simulink model "Four_Robots_Swarm"  (R2021a)
settings: Solver=FixedStepAuto  StartTime=0.0  StopTime=inf  FixedStep=0.01  RelTol=1e-3  EnableMultiTasking=on
model workspace (MAT data in the model file):
  SL_ROS_VariableLengthArrays_MaxSizes : object (value not decoded)
undefined symbols (not defined in the file or in its folder): Angular, DistanceGoal, L, Linear, PP, theta, Way1, Way2, Way3, Way4
libraries: robotlib x17, robotalgslib x8
(part 2 of 2)

== system Four_Robots_Swarm/Swarm/TurtleBot2/ Avoiding Obstacles/Path Following ==
  SteeringDirection : Inport
  AngularVelocity : Inport  Port=2
  Action Port : ActionPort  ActionPortLabel=else
  Compute Angular Velocity : MATLAB Function  TreatAsAtomicUnit=on
  Constant : Constant  Value=0
  MaxAngularVelocity : Constant  Value=1.82
  Subtract : Sum  Inputs=+-
  dV : Outport  VectorParamsAs1DForOutWhenUnconnected=off
  dW : Outport  Port=2  VectorParamsAs1DForOutWhenUnconnected=off
  wires:
  AngularVelocity/1 -> Subtract/2
  Compute Angular Velocity/1(w) -> Subtract/1
  Subtract/1 -> dW/1
  SteeringDirection/1 -> Compute Angular Velocity/1(steeringDir)
  MaxAngularVelocity/1 -> Compute Angular Velocity/2(wMax)
  Constant/1 -> dV/1

== system Four_Robots_Swarm/Swarm/TurtleBot2/ Avoiding Obstacles/Recovery ==
  LinearVelocity : Inport
  AngularVelocity_comp : Inport  Port=2
  AngularVelocity : Inport  Port=3
  Action Port : ActionPort  ActionPortLabel=if(u1 == 1)
  Gain : Gain  Gain=-1
  Subtract : Sum  Inputs=|+-
  dV : Outport  VectorParamsAs1DForOutWhenUnconnected=off
  dW : Outport  Port=2  VectorParamsAs1DForOutWhenUnconnected=off
  wires:
  Subtract/1 -> dW/1
  AngularVelocity/1 -> Subtract/2
  Gain/1 -> dV/1
  LinearVelocity/1 -> Gain/1
  AngularVelocity_comp/1 -> Subtract/1

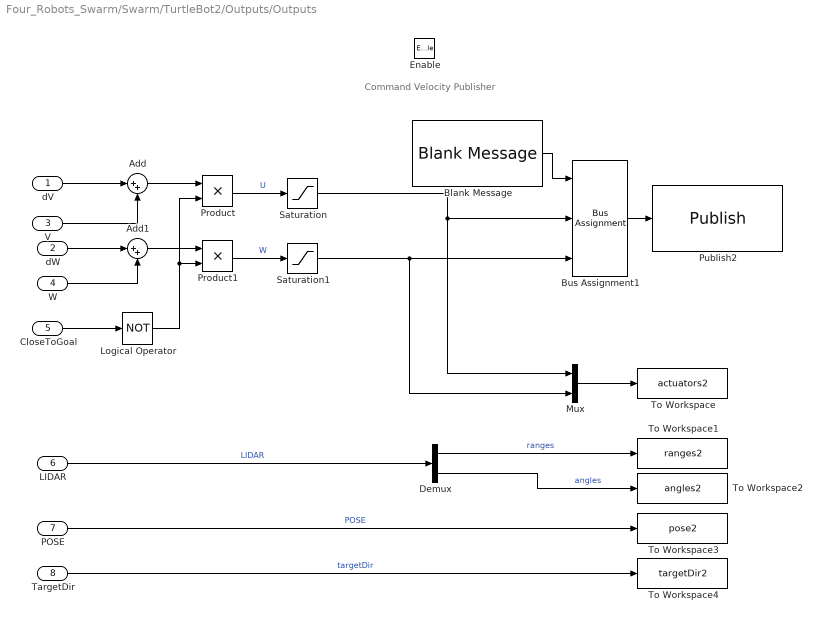
== system Four_Robots_Swarm/Swarm/TurtleBot2/Outputs/Outputs ==
  note: Command Velocity Publisher
  dV : Inport
  dW : Inport  Port=2
  V : Inport  Port=3
  W : Inport  Port=4
  CloseToGoal : Inport  Port=5
  LIDAR : Inport  Port=6
  POSE : Inport  Port=7
  TargetDir : Inport  Port=8
  Enable : EnablePort
  Add : Sum  Inputs=|++
  Add1 : Sum  Inputs=|++
  Blank Message : robotlib/Blank Message  messageClass=Message  entityType=geometry_msgs/Twist  messageType=geometry_msgs/Twist  SampleTime=inf  legacyBusStruct=off
  Bus Assignment1 : BusAssignment  DialogController=Simulink.DDGSource_BusAssignment  AssignedSignals=Linear.X,Angular.Z
  Demux : Demux  Outputs=2
  Logical Operator : Logic  Operator=NOT  AllPortsSameDT=off  OutDataTypeStr=boolean
  Mux : Mux  Inputs=2
  Product : Product
  Product1 : Product
  Publish2 : robotlib/Publish  topicSource=Select from ROS network  topic=/robot2/cmd_vel  messageType=geometry_msgs/Twist  legacyBusStruct=off  messageQueueLength=105
  Saturation : Saturate  UpperLimit=PP.DesiredLinearVelocity  LowerLimit=-PP.DesiredLinearVelocity
  Saturation1 : Saturate  UpperLimit=PP.MaxAngularVelocity  LowerLimit=-PP.MaxAngularVelocity
  To Workspace : ToWorkspace  VariableName=actuators2  SaveFormat=Structure With Time  SampleTime=0.01
      settings: Decimation=2
  To Workspace1 : ToWorkspace  VariableName=ranges2  SaveFormat=Structure With Time  SampleTime=0.01
      settings: Decimation=2
  To Workspace2 : ToWorkspace  VariableName=angles2  SaveFormat=Structure With Time  SampleTime=0.01
      settings: Decimation=2
  To Workspace3 : ToWorkspace  VariableName=pose2  SaveFormat=Structure With Time  SampleTime=0.01
      settings: Decimation=2
  To Workspace4 : ToWorkspace  VariableName=targetDir2  SaveFormat=Structure With Time  SampleTime=0.01
      settings: Decimation=2
  wires:
  V/1 -> Add/2
  W/1 -> Add1/2
  dV/1 -> Add/1
  dW/1 -> Add1/1
  CloseToGoal/1 -> Logical Operator/1
  Add/1 -> Product/1
  Add1/1 -> Product1/1
  Blank Message/1 -> Bus Assignment1/1
  Bus Assignment1/1 -> Publish2/1
  Logical Operator/1 -> Product1/2, Product/2
  Mux/1 -> To Workspace/1
  Product/1 -> Saturation/1  "U"
  Saturation/1 -> Mux/1, Bus Assignment1/2
  Product1/1 -> Saturation1/1  "W"
  Saturation1/1 -> Mux/2, Bus Assignment1/3
  TargetDir/1 -> To Workspace4/1  "targetDir"
  Demux/2 -> To Workspace2/1  "angles"
  LIDAR/1 -> Demux/1  "LIDAR"
  POSE/1 -> To Workspace3/1  "POSE"
  Demux/1 -> To Workspace1/1  "ranges"

== system Four_Robots_Swarm/Swarm/TurtleBot2/Subsystem/Enabled Subsystem ==
  WAY : Inport
  DATA : Inport  Port=2
  Enable : EnablePort
  MATLAB Function2 : MATLAB Function  TreatAsAtomicUnit=on
  I : Outport
  wires:
  WAY/1 -> MATLAB Function2/1(WAY)
  DATA/1 -> MATLAB Function2/2(DATA)
  MATLAB Function2/1(I) -> I/1

== system Four_Robots_Swarm/Swarm/TurtleBot3/ Avoiding Obstacles/Path Following ==
  SteeringDirection : Inport
  AngularVelocity : Inport  Port=2
  Action Port : ActionPort  ActionPortLabel=else
  Compute Angular Velocity : MATLAB Function  TreatAsAtomicUnit=on
  Constant : Constant  Value=0
  MaxAngularVelocity : Constant  Value=1.82
  Subtract : Sum  Inputs=+-
  dV : Outport  VectorParamsAs1DForOutWhenUnconnected=off
  dW : Outport  Port=2  VectorParamsAs1DForOutWhenUnconnected=off
  wires:
  AngularVelocity/1 -> Subtract/2
  Compute Angular Velocity/1(w) -> Subtract/1
  Subtract/1 -> dW/1
  SteeringDirection/1 -> Compute Angular Velocity/1(steeringDir)
  MaxAngularVelocity/1 -> Compute Angular Velocity/2(wMax)
  Constant/1 -> dV/1

== system Four_Robots_Swarm/Swarm/TurtleBot3/ Avoiding Obstacles/Recovery ==
  LinearVelocity : Inport
  AngularVelocity_comp : Inport  Port=2
  AngularVelocity : Inport  Port=3
  Action Port : ActionPort  ActionPortLabel=if(u1 == 1)
  Gain : Gain  Gain=-1
  Subtract : Sum  Inputs=|+-
  dV : Outport  VectorParamsAs1DForOutWhenUnconnected=off
  dW : Outport  Port=2  VectorParamsAs1DForOutWhenUnconnected=off
  wires:
  Subtract/1 -> dW/1
  AngularVelocity/1 -> Subtract/2
  Gain/1 -> dV/1
  LinearVelocity/1 -> Gain/1
  AngularVelocity_comp/1 -> Subtract/1

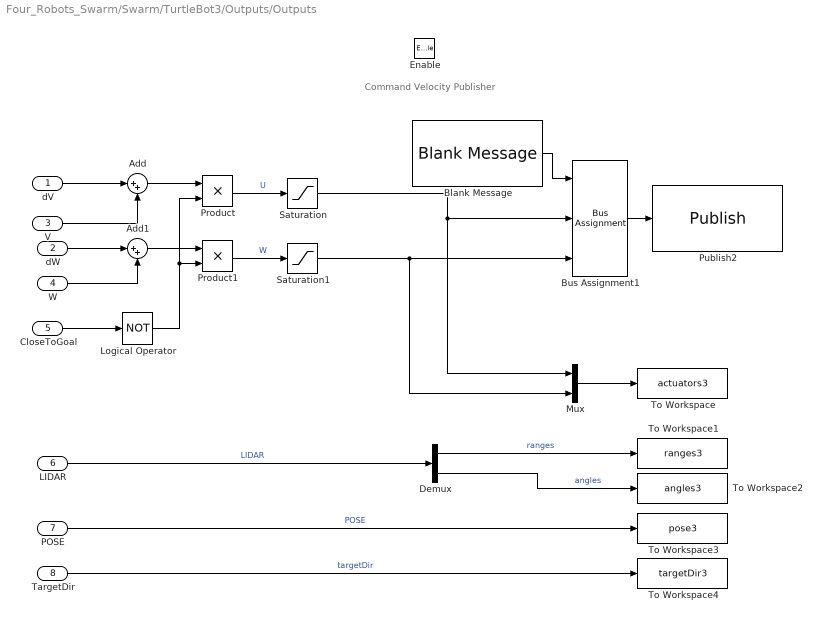
== system Four_Robots_Swarm/Swarm/TurtleBot3/Outputs/Outputs ==
  note: Command Velocity Publisher
  dV : Inport
  dW : Inport  Port=2
  V : Inport  Port=3
  W : Inport  Port=4
  CloseToGoal : Inport  Port=5
  LIDAR : Inport  Port=6
  POSE : Inport  Port=7
  TargetDir : Inport  Port=8
  Enable : EnablePort
  Add : Sum  Inputs=|++
  Add1 : Sum  Inputs=|++
  Blank Message : robotlib/Blank Message  messageClass=Message  entityType=geometry_msgs/Twist  messageType=geometry_msgs/Twist  SampleTime=inf  legacyBusStruct=off
  Bus Assignment1 : BusAssignment  DialogController=Simulink.DDGSource_BusAssignment  AssignedSignals=Linear.X,Angular.Z
  Demux : Demux  Outputs=2
  Logical Operator : Logic  Operator=NOT  AllPortsSameDT=off  OutDataTypeStr=boolean
  Mux : Mux  Inputs=2
  Product : Product
  Product1 : Product
  Publish2 : robotlib/Publish  topicSource=Select from ROS network  topic=/robot3/cmd_vel  messageType=geometry_msgs/Twist  legacyBusStruct=off  messageQueueLength=105
  Saturation : Saturate  UpperLimit=PP.DesiredLinearVelocity  LowerLimit=-PP.DesiredLinearVelocity
  Saturation1 : Saturate  UpperLimit=PP.MaxAngularVelocity  LowerLimit=-PP.MaxAngularVelocity
  To Workspace : ToWorkspace  VariableName=actuators3  SaveFormat=Structure With Time  SampleTime=0.01
      settings: Decimation=2
  To Workspace1 : ToWorkspace  VariableName=ranges3  SaveFormat=Structure With Time  SampleTime=0.01
      settings: Decimation=2
  To Workspace2 : ToWorkspace  VariableName=angles3  SaveFormat=Structure With Time  SampleTime=0.01
      settings: Decimation=2
  To Workspace3 : ToWorkspace  VariableName=pose3  SaveFormat=Structure With Time  SampleTime=0.01
      settings: Decimation=2
  To Workspace4 : ToWorkspace  VariableName=targetDir3  SaveFormat=Structure With Time  SampleTime=0.01
      settings: Decimation=2
  wires:
  V/1 -> Add/2
  W/1 -> Add1/2
  dV/1 -> Add/1
  dW/1 -> Add1/1
  CloseToGoal/1 -> Logical Operator/1
  Add/1 -> Product/1
  Add1/1 -> Product1/1
  Blank Message/1 -> Bus Assignment1/1
  Bus Assignment1/1 -> Publish2/1
  Logical Operator/1 -> Product1/2, Product/2
  Mux/1 -> To Workspace/1
  Product/1 -> Saturation/1  "U"
  Saturation/1 -> Mux/1, Bus Assignment1/2
  Product1/1 -> Saturation1/1  "W"
  Saturation1/1 -> Mux/2, Bus Assignment1/3
  TargetDir/1 -> To Workspace4/1  "targetDir"
  Demux/2 -> To Workspace2/1  "angles"
  LIDAR/1 -> Demux/1  "LIDAR"
  POSE/1 -> To Workspace3/1  "POSE"
  Demux/1 -> To Workspace1/1  "ranges"

== system Four_Robots_Swarm/Swarm/TurtleBot3/Subsystem/Enabled Subsystem ==
  WAY : Inport
  DATA : Inport  Port=2
  Enable : EnablePort
  MATLAB Function2 : MATLAB Function  TreatAsAtomicUnit=on
  I : Outport
  wires:
  WAY/1 -> MATLAB Function2/1(WAY)
  DATA/1 -> MATLAB Function2/2(DATA)
  MATLAB Function2/1(I) -> I/1

== system Four_Robots_Swarm/Swarm/TurtleBot4/ Avoiding Obstacles/Path Following ==
  SteeringDirection : Inport
  AngularVelocity : Inport  Port=2
  Action Port : ActionPort  ActionPortLabel=else
  Compute Angular Velocity : MATLAB Function  TreatAsAtomicUnit=on
  Constant : Constant  Value=0
  MaxAngularVelocity : Constant  Value=1.82
  Subtract : Sum  Inputs=+-
  dV : Outport  VectorParamsAs1DForOutWhenUnconnected=off
  dW : Outport  Port=2  VectorParamsAs1DForOutWhenUnconnected=off
  wires:
  AngularVelocity/1 -> Subtract/2
  Compute Angular Velocity/1(w) -> Subtract/1
  Subtract/1 -> dW/1
  SteeringDirection/1 -> Compute Angular Velocity/1(steeringDir)
  MaxAngularVelocity/1 -> Compute Angular Velocity/2(wMax)
  Constant/1 -> dV/1

== system Four_Robots_Swarm/Swarm/TurtleBot4/ Avoiding Obstacles/Recovery ==
  LinearVelocity : Inport
  AngularVelocity_comp : Inport  Port=2
  AngularVelocity : Inport  Port=3
  Action Port : ActionPort  ActionPortLabel=if(u1 == 1)
  Gain : Gain  Gain=-1
  Subtract : Sum  Inputs=|+-
  dV : Outport  VectorParamsAs1DForOutWhenUnconnected=off
  dW : Outport  Port=2  VectorParamsAs1DForOutWhenUnconnected=off
  wires:
  Subtract/1 -> dW/1
  AngularVelocity/1 -> Subtract/2
  Gain/1 -> dV/1
  LinearVelocity/1 -> Gain/1
  AngularVelocity_comp/1 -> Subtract/1

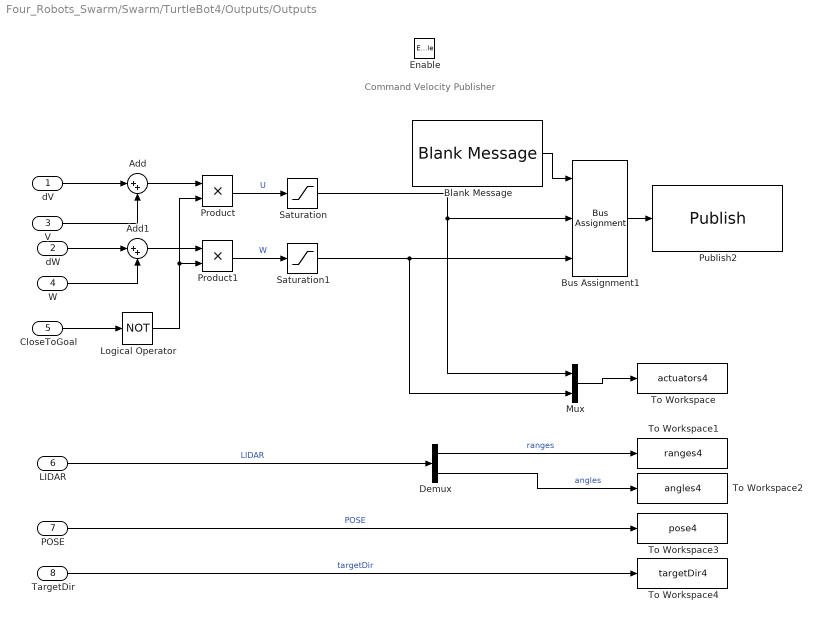
== system Four_Robots_Swarm/Swarm/TurtleBot4/Outputs/Outputs ==
  note: Command Velocity Publisher
  dV : Inport
  dW : Inport  Port=2
  V : Inport  Port=3
  W : Inport  Port=4
  CloseToGoal : Inport  Port=5
  LIDAR : Inport  Port=6
  POSE : Inport  Port=7
  TargetDir : Inport  Port=8
  Enable : EnablePort
  Add : Sum  Inputs=|++
  Add1 : Sum  Inputs=|++
  Blank Message : robotlib/Blank Message  messageClass=Message  entityType=geometry_msgs/Twist  messageType=geometry_msgs/Twist  SampleTime=inf  legacyBusStruct=off
  Bus Assignment1 : BusAssignment  DialogController=Simulink.DDGSource_BusAssignment  AssignedSignals=Linear.X,Angular.Z
  Demux : Demux  Outputs=2
  Logical Operator : Logic  Operator=NOT  AllPortsSameDT=off  OutDataTypeStr=boolean
  Mux : Mux  Inputs=2
  Product : Product
  Product1 : Product
  Publish2 : robotlib/Publish  topicSource=Select from ROS network  topic=/robot4/cmd_vel  messageType=geometry_msgs/Twist  legacyBusStruct=off  messageQueueLength=105
  Saturation : Saturate  UpperLimit=PP.DesiredLinearVelocity  LowerLimit=-PP.DesiredLinearVelocity
  Saturation1 : Saturate  UpperLimit=PP.MaxAngularVelocity  LowerLimit=-PP.MaxAngularVelocity
  To Workspace : ToWorkspace  VariableName=actuators4  SaveFormat=Structure With Time  SampleTime=0.01
      settings: Decimation=2
  To Workspace1 : ToWorkspace  VariableName=ranges4  SaveFormat=Structure With Time  SampleTime=0.01
      settings: Decimation=2
  To Workspace2 : ToWorkspace  VariableName=angles4  SaveFormat=Structure With Time  SampleTime=0.01
      settings: Decimation=2
  To Workspace3 : ToWorkspace  VariableName=pose4  SaveFormat=Structure With Time  SampleTime=0.01
      settings: Decimation=2
  To Workspace4 : ToWorkspace  VariableName=targetDir4  SaveFormat=Structure With Time  SampleTime=0.01
      settings: Decimation=2
  wires:
  V/1 -> Add/2
  W/1 -> Add1/2
  dV/1 -> Add/1
  dW/1 -> Add1/1
  CloseToGoal/1 -> Logical Operator/1
  Add/1 -> Product/1
  Add1/1 -> Product1/1
  Blank Message/1 -> Bus Assignment1/1
  Bus Assignment1/1 -> Publish2/1
  Logical Operator/1 -> Product1/2, Product/2
  Mux/1 -> To Workspace/1
  Product/1 -> Saturation/1  "U"
  Saturation/1 -> Mux/1, Bus Assignment1/2
  Product1/1 -> Saturation1/1  "W"
  Saturation1/1 -> Mux/2, Bus Assignment1/3
  TargetDir/1 -> To Workspace4/1  "targetDir"
  Demux/2 -> To Workspace2/1  "angles"
  LIDAR/1 -> Demux/1  "LIDAR"
  POSE/1 -> To Workspace3/1  "POSE"
  Demux/1 -> To Workspace1/1  "ranges"

== system Four_Robots_Swarm/Swarm/TurtleBot4/Subsystem/Enabled Subsystem ==
  WAY : Inport
  DATA : Inport  Port=2
  Enable : EnablePort
  MATLAB Function2 : MATLAB Function  TreatAsAtomicUnit=on
  I : Outport
  wires:
  WAY/1 -> MATLAB Function2/1(WAY)
  DATA/1 -> MATLAB Function2/2(DATA)
  MATLAB Function2/1(I) -> I/1

== matlab function Four_Robots_Swarm/Swarm/TurtleBot2/Inputs/quad2eul ==
  data: X input; Yaw output; Y input; Z input; W input
function Yaw = quat2eulBlk(X, Y, Z, W)
%#codegen

eularAngles = quat2eul([W, X, Y, Z]);
Yaw = eularAngles(1);

== matlab function Four_Robots_Swarm/Swarm/TurtleBot4/ Avoiding Obstacles/Path Following/Compute Angular Velocity ==
  data: steeringDir input; w output; wMax input
function w = exampleHelperComputeAngularVelocity(steeringDir, wMax)
%EXAMPLEHELPERCOMPUTEANGULARVELOCITY Compute angular velocity
%   W = exampleHelperComputeAngularVelocity(STEERINGDIR)
%   returns the angular velocity W for a differential drive robot in radians
%   per second for a given steering direction STEERINGDIR in the robot's
%   coordinate frame in radians.
%
%   W = exampleHelperComputeAngularVelocity(STEERINGDIR, WMAX)
%   returns the angular velocity W for a differential drive robot in radians
%   per second for a given steering direction STEERINGDIR in the robot's
%   coordinate frame in radians and maximum angular velocity WMAX in
%   radians per second. The output angular velocity is saturated based on
%   the WMAX.
%
%   Example:
%       
%       w = exampleHelperComputeAngularVelocity(0.2, 1);

% Copyright 2015 The MathWorks, Inc.

%#codegen
%#ok<*EMCA>

% Allow variable input arguments
if nargin == 1   
    wMax = inf;
end

validateattributes(steeringDir, {'double'},{'real'},...
    'exampleHelperComputeAngularVelocity', 'STEERINGDIR', 1);
validateattributes(wMax, {'double'},{'real', 'positive'},...
    'exampleHelperComputeAngularVelocity', 'WMAX', 2);

% Computing in robot's coordinate frame
curPose = [0 0 0];

% The following computation is similar to robotics.PurePursuit
lookaheadPoint = [cos(steeringDir), sin(steeringDir)];
slope = atan2((lookaheadPoint(2) - curPose(2)), ...
    (lookaheadPoint(1) - curPose(1)));
alpha = angdiff(curPose(3), slope);

% Angular velocity command for a differential drive robot is
% equal to the desired curvature to be followed by the robot.

w = (2*sin(alpha));

% Pick a constant rotation when robot is facing in the opposite
% direction of the path
if abs(abs(alpha) - pi) < 1e-12
    w = sign(w)*1;
end

if abs(w) > wMax
    w = sign(w)*wMax;
end

end

== matlab function Four_Robots_Swarm/Swarm/TurtleBot4/ Path following/ Extract Goal ==
  data: Waypoints input; Goal output
function Goal = extractGoal(Waypoints)
%#codegen
b = isnan(Waypoints);
[rows,~] = find(b);
ridx = setdiff(1:size(Waypoints,1), sort(rows));
Goal = [Waypoints(ridx(end), 1) Waypoints(ridx(end), 2)];

== matlab function Four_Robots_Swarm/Swarm/TurtleBot4/Inputs/MATLAB Function ==
  data: LaserScanMsg input; Ranges output; Angles output
function [Ranges, Angles] = ExtractRangeData(LaserScanMsg)
%#codegen

% Extract Range information
Ranges = double(LaserScanMsg.Ranges);

% Construct Angles vector using AngleMin and AngleIncrement from sensor
% reading.
angMin = double(LaserScanMsg.AngleMin);
angIncrement = double(LaserScanMsg.AngleIncrement);

numReadings = numel(Ranges);
rawAngles = angMin + (0:numReadings-1)' * angIncrement;

% Wrap the angles to the (-pi,pi] interval.
Angles = robotics.internal.wrapToPi(double(rawAngles));

== matlab function Four_Robots_Swarm/Swarm/TurtleBot3/Inputs/quad2eul ==
  data: X input; Yaw output; Y input; Z input; W input
function Yaw = quat2eulBlk(X, Y, Z, W)
%#codegen

eularAngles = quat2eul([W, X, Y, Z]);
Yaw = eularAngles(1);

== matlab function Four_Robots_Swarm/Swarm/TurtleBot4/Inputs/quad2eul ==
  data: X input; Yaw output; Y input; Z input; W input
function Yaw = quat2eulBlk(X, Y, Z, W)
%#codegen

eularAngles = quat2eul([W, X, Y, Z]);
Yaw = eularAngles(1);

== matlab function Four_Robots_Swarm/Swarm/TurtleBot1/MATLAB Function ==
  data: DATA input; way output; i input
function way = fcn(DATA,i)
n=4;
POSE1=DATA(1:3);
POSE2=DATA(4:6);
POSE3=DATA(7:9);
POSE4=DATA(10:12);

POSES={POSE1,POSE2,POSE3,POSE4};
POSEi=POSES{i}; %determino el i robot (mismo algoritmo todos los robots)
POSESn={POSEi,POSE2,POSE3,POSE4};

%% Cálculo distancias robots
%di_i no se calcula
% di_2=sqrt((POSEi(1)-POSE2(1))^2+(POSEi(2)-POSE2(2))^2);
d=zeros(1,n-1);
for j=2:n
  POSEj=POSESn{j}; 
  d(j-1)=sqrt((POSEi(1)-POSEj(1))^2+(POSEj(2)-POSEj(2))^2);  
end
%% AggregationProcedure
%determinar limites
[~,prox]=min(d);
POSEprox=POSESn{prox+1};% para sacar la posición del robot mas cercano
[~,far]=max(d);
POSEfar=POSESn{far+1};% para sacar la posición del robot mas lejano
% calculo punto deseado
xd=(POSEi(1)+POSEprox(1)+POSEfar(1))/3;
yd=(POSEi(2)+POSEprox(2)+POSEfar(2))/3;
%envio way para pure_pursuit
way=[POSEi(1) POSEi(2);xd yd];

== matlab function Four_Robots_Swarm/Swarm/TurtleBot3/MATLAB Function1 ==
  data: DATA input; way output; i input
function way = fcn(DATA,i)
n=4;
POSE1=DATA(1:3);
POSE2=DATA(4:6);
POSE3=DATA(7:9);
POSE4=DATA(10:12);

POSES={POSE1,POSE2,POSE3,POSE4};
POSEi=POSES{i}; %determino el i robot (mismo algoritmo todos los robots)
POSESn={POSEi,POSE1,POSE2,POSE4};

%% Cálculo distancias robots
%di_i no se calcula
% di_2=sqrt((POSEi(1)-POSE2(1))^2+(POSEi(2)-POSE2(2))^2);
d=zeros(1,n-1);
for j=2:n
  POSEj=POSESn{j}; 
  d(j-1)=sqrt((POSEi(1)-POSEj(1))^2+(POSEj(2)-POSEj(2))^2);  
end
%% AggregationProcedure
%determinar limites
[~,prox]=min(d);
POSEprox=POSESn{prox+1};% para sacar la posición del robot mas cercano
[~,far]=max(d);
POSEfar=POSESn{far+1};% para sacar la posición del robot mas lejano
% calculo punto deseado
xd=(POSEi(1)+POSEprox(1)+POSEfar(1))/3;
yd=(POSEi(2)+POSEprox(2)+POSEfar(2))/3;
%envio way para pure_pursuit
way=[POSEi(1) POSEi(2);xd yd];

== matlab function Four_Robots_Swarm/Swarm/TurtleBot4/MATLAB Function1 ==
  data: DATA input; way output; i input
function way = fcn(DATA,i)
n=4;
POSE1=DATA(1:3);
POSE2=DATA(4:6);
POSE3=DATA(7:9);
POSE4=DATA(10:12);

POSES={POSE1,POSE2,POSE3,POSE4};
POSEi=POSES{i}; %determino el i robot (mismo algoritmo todos los robots)
POSESn={POSEi,POSE1,POSE3,POSE4};

%% Cálculo distancias robots
%di_i no se calcula
% di_2=sqrt((POSEi(1)-POSE2(1))^2+(POSEi(2)-POSE2(2))^2);
d=zeros(1,n-1);
for j=2:n
  POSEj=POSESn{j}; 
  d(j-1)=sqrt((POSEi(1)-POSEj(1))^2+(POSEj(2)-POSEj(2))^2);  
end
%% AggregationProcedure
%determinar limites
[~,prox]=min(d);
POSEprox=POSESn{prox+1};% para sacar la posición del robot mas cercano
[~,far]=max(d);
POSEfar=POSESn{far+1};% para sacar la posición del robot mas lejano
% calculo punto deseado
xd=(POSEi(1)+POSEprox(1)+POSEfar(1))/3;
yd=(POSEi(2)+POSEprox(2)+POSEfar(2))/3;
%envio way para pure_pursuit
way=[POSEi(1) POSEi(2);xd yd];

== matlab function Four_Robots_Swarm/Joystick/Triggered Subsystem/MATLAB Function1 ==
  data: axes input; buttons input; x_ax output; y_ax output; A output; B output; X output; Y output
function [x_ax,y_ax,A,B,X,Y] = fcn(axes, buttons)
x_ax=axes(1);
y_ax=axes(2);
A=buttons(1);
B=buttons(2);
X=buttons(3);
Y=buttons(4);

== matlab function Four_Robots_Swarm/Swarm/TurtleBot1/Subsystem/Enabled Subsystem/MATLAB Function2 ==
  data: WAY input; DATA input; I output
function I  = fcn(WAY,DATA)
n=4;
POSE1=DATA(1:3);
POSE2=DATA(4:6);
POSE3=DATA(7:9);
POSE4=DATA(10:12);



POSES={POSE1,POSE2,POSE3,POSE4};

%% Cálculo distancias robots- origen trayectoria
xway=WAY(1,1);
yway=WAY(1,2);
d=zeros(1,n);
for j=1:n
  POSEj=POSES{j};  
  d(j)=sqrt((xway-POSEj(1))^2+(yway-POSEj(2))^2);  
end
%% Determino orden robots
[~,I]=sort(d);

== matlab function Four_Robots_Swarm/Swarm/TurtleBot1/Subsystem/MATLAB Function1 ==
  data: WAY input; DATA input; way output double; i input; I input; l input; theta_n input
function way = fcn(WAY,DATA,i,I,l,theta_n)
n=4;
kw=size(WAY,1);
POSE1=DATA(1:3);
POSE2=DATA(4:6);
POSE3=DATA(7:9);
POSE4=DATA(10:12);

POSES={POSE1,POSE2,POSE3,POSE4};
POSEi=POSES{i}; %determino el i robot (mismo algoritmo todos los robots)

POSEsorted=POSES;
for k=1:n
    POSEsorted{k}=POSES{I(k)};  
end 

%% Flocking
POSE_lead=POSEsorted{1};
x=zeros(1,n);
y=zeros(1,n);
theta=zeros(1,n);

x(1)=POSE_lead(1);
y(1)=POSE_lead(2);
theta(1)=POSE_lead(3);
xd=x(1);
yd=y(1);

for k=2:n
    POSE_current=POSEsorted{k};
    theta(k)=POSE_current(3);
    
    x(k)=x(k-1)+l*sin(theta(k-1)-theta_n);
    y(k)=y(k-1)+l*cos(theta(k-1)-theta_n);
end    
if i==I(1)
   way=WAY;
else
   for k=2:n
       if I(k)==i
          xd=x(k);
          yd=y(k);
          break;
       else
          xd=xd;
          yd=yd;
       end    
   end    
    %envio way para pure_pursuit
   way=WAY; 
   for k=1:kw
      if k<kw
        way(k,1)= POSEi(1);
        way(k,2)= POSEi(2);
      else
        way(k,1)= xd;
        way(k,2)= yd;   
      end
   end
end

== matlab function Four_Robots_Swarm/Swarm/TurtleBot1/selector ==
  data: sel input; way output; way_swap input; way_aggre input; way_flocking input
function way = fcn(sel,way_swap,way_aggre,way_flocking)
if sel==0
    way=way_swap;
elseif sel==1
    way=way_aggre;
elseif sel==2
    way=way_flocking;   
else
    way=way_swap;    
end

== matlab function Four_Robots_Swarm/Joystick/Triggered Subsystem/MATLAB Function ==
  data: x input; Pf output; y input
function Pf = fcn(x,y)
Pf= [x y];

== matlab function Four_Robots_Swarm/Swarm/TurtleBot1/MATLAB Function1 ==
  data: p_i input; p_f input; way output
function way = fcn(p_i,p_f)
way=[p_i(1),p_i(2) ;p_f(1),p_f(2)];

== matlab function Four_Robots_Swarm/Swarm/TurtleBot2/MATLAB Function1 ==
  data: DATA input; way output; i input
function way = fcn(DATA,i)
n=4;
POSE1=DATA(1:3);
POSE2=DATA(4:6);
POSE3=DATA(7:9);
POSE4=DATA(10:12);

POSES={POSE1,POSE2,POSE3,POSE4};
POSEi=POSES{i}; %determino el i robot (mismo algoritmo todos los robots)
POSESn={POSEi,POSE1,POSE3,POSE4};

%% Cálculo distancias robots
%di_i no se calcula
% di_2=sqrt((POSEi(1)-POSE2(1))^2+(POSEi(2)-POSE2(2))^2);
d=zeros(1,n-1);
for j=2:n
  POSEj=POSESn{j}; 
  d(j-1)=sqrt((POSEi(1)-POSEj(1))^2+(POSEj(2)-POSEj(2))^2);  
end
%% AggregationProcedure
%determinar limites
[~,prox]=min(d);
POSEprox=POSESn{prox+1};% para sacar la posición del robot mas cercano
[~,far]=max(d);
POSEfar=POSESn{far+1};% para sacar la posición del robot mas lejano
% calculo punto deseado
xd=(POSEi(1)+POSEprox(1)+POSEfar(1))/3;
yd=(POSEi(2)+POSEprox(2)+POSEfar(2))/3;
%envio way para pure_pursuit
way=[POSEi(1) POSEi(2);xd yd];

== matlab function Four_Robots_Swarm/Swarm/TurtleBot3/ Avoiding Obstacles/Path Following/Compute Angular Velocity ==
  data: steeringDir input; w output; wMax input
function w = exampleHelperComputeAngularVelocity(steeringDir, wMax)
%EXAMPLEHELPERCOMPUTEANGULARVELOCITY Compute angular velocity
%   W = exampleHelperComputeAngularVelocity(STEERINGDIR)
%   returns the angular velocity W for a differential drive robot in radians
%   per second for a given steering direction STEERINGDIR in the robot's
%   coordinate frame in radians.
%
%   W = exampleHelperComputeAngularVelocity(STEERINGDIR, WMAX)
%   returns the angular velocity W for a differential drive robot in radians
%   per second for a given steering direction STEERINGDIR in the robot's
%   coordinate frame in radians and maximum angular velocity WMAX in
%   radians per second. The output angular velocity is saturated based on
%   the WMAX.
%
%   Example:
%       
%       w = exampleHelperComputeAngularVelocity(0.2, 1);

% Copyright 2015 The MathWorks, Inc.

%#codegen
%#ok<*EMCA>

% Allow variable input arguments
if nargin == 1   
    wMax = inf;
end

validateattributes(steeringDir, {'double'},{'real'},...
    'exampleHelperComputeAngularVelocity', 'STEERINGDIR', 1);
validateattributes(wMax, {'double'},{'real', 'positive'},...
    'exampleHelperComputeAngularVelocity', 'WMAX', 2);

% Computing in robot's coordinate frame
curPose = [0 0 0];

% The following computation is similar to robotics.PurePursuit
lookaheadPoint = [cos(steeringDir), sin(steeringDir)];
slope = atan2((lookaheadPoint(2) - curPose(2)), ...
    (lookaheadPoint(1) - curPose(1)));
alpha = angdiff(curPose(3), slope);

% Angular velocity command for a differential drive robot is
% equal to the desired curvature to be followed by the robot.

w = (2*sin(alpha));

% Pick a constant rotation when robot is facing in the opposite
% direction of the path
if abs(abs(alpha) - pi) < 1e-12
    w = sign(w)*1;
end

if abs(w) > wMax
    w = sign(w)*wMax;
end

end

== matlab function Four_Robots_Swarm/Swarm/TurtleBot2/MATLAB Function2 ==
  data: p_i input; p_f input; way output
function way = fcn(p_i,p_f)
way=[p_i(1),p_i(2) ;p_f(1),p_f(2)];

== matlab function Four_Robots_Swarm/Swarm/TurtleBot2/Subsystem/Enabled Subsystem/MATLAB Function2 ==
  data: WAY input; DATA input; I output
function I  = fcn(WAY,DATA)
n=4;
POSE1=DATA(1:3);
POSE2=DATA(4:6);
POSE3=DATA(7:9);
POSE4=DATA(10:12);

POSES={POSE1,POSE2,POSE3,POSE4};

%% Cálculo distancias robots- origen trayectoria
xway=WAY(1,1);
yway=WAY(1,2);
d=zeros(1,n);
for j=1:n
  POSEj=POSES{j};  
  d(j)=sqrt((xway-POSEj(1))^2+(yway-POSEj(2))^2);  
end
%% Determino orden robots
[~,I]=sort(d);

== matlab function Four_Robots_Swarm/Swarm/TurtleBot2/Subsystem/MATLAB Function1 ==
  data: WAY input; DATA input; way output double; i input; I input; l input; theta_n input
function way = fcn(WAY,DATA,i,I,l,theta_n)
n=4;
kw=size(WAY,1);
POSE1=DATA(1:3);
POSE2=DATA(4:6);
POSE3=DATA(7:9);
POSE4=DATA(10:12);

POSES={POSE1,POSE2,POSE3,POSE4};
POSEi=POSES{i}; %determino el i robot (mismo algoritmo todos los robots)

POSEsorted=POSES;
for k=1:n
    POSEsorted{k}=POSES{I(k)};  
end 

%% Flocking
POSE_lead=POSEsorted{1};
x=zeros(1,n);
y=zeros(1,n);
theta=zeros(1,n);

x(1)=POSE_lead(1);
y(1)=POSE_lead(2);
theta(1)=POSE_lead(3);
xd=x(1);
yd=y(1);

for k=2:n
    POSE_current=POSEsorted{k};
    theta(k)=POSE_current(3);
    
    x(k)=x(k-1)+l*sin(theta(k-1)-theta_n);
    y(k)=y(k-1)+l*cos(theta(k-1)-theta_n);
end    
if i==I(1)
   way=WAY;
else
   for k=2:n
       if I(k)==i
          xd=x(k);
          yd=y(k);
          break;
       else
          xd=xd;
          yd=yd;
       end    
   end    
    %envio way para pure_pursuit
   way=WAY; 
   for k=1:kw
      if k<kw
        way(k,1)= POSEi(1);
        way(k,2)= POSEi(2);
      else
        way(k,1)= xd;
        way(k,2)= yd;   
      end
   end
end

== matlab function Four_Robots_Swarm/Swarm/TurtleBot2/selector ==
  data: sel input; way output; way_swap input; way_aggre input; way_flocking input
function way = fcn(sel,way_swap,way_aggre,way_flocking)
if sel==0
    way=way_swap;
elseif sel==1
    way=way_aggre;
elseif sel==2
    way=way_flocking;   
else
    way=way_swap;    
end

== matlab function Four_Robots_Swarm/Swarm/TurtleBot3/MATLAB Function2 ==
  data: p_i input; p_f input; way output
function way = fcn(p_i,p_f)
way=[p_i(1),p_i(2) ;p_f(1),p_f(2)];

== matlab function Four_Robots_Swarm/Swarm/TurtleBot3/Subsystem/Enabled Subsystem/MATLAB Function2 ==
  data: WAY input; DATA input; I output
function I  = fcn(WAY,DATA)
n=4;
POSE1=DATA(1:3);
POSE2=DATA(4:6);
POSE3=DATA(7:9);
POSE4=DATA(10:12);

POSES={POSE1,POSE2,POSE3,POSE4};

%% Cálculo distancias robots- origen trayectoria
xway=WAY(1,1);
yway=WAY(1,2);
d=zeros(1,n);
for j=1:n
  POSEj=POSES{j};  
  d(j)=sqrt((xway-POSEj(1))^2+(yway-POSEj(2))^2);  
end
%% Determino orden robots
[~,I]=sort(d);

== matlab function Four_Robots_Swarm/Swarm/TurtleBot3/Subsystem/MATLAB Function1 ==
  data: WAY input; DATA input; way output double; i input; I input; l input; theta_n input
function way = fcn(WAY,DATA,i,I,l,theta_n)
n=4;
kw=size(WAY,1);
POSE1=DATA(1:3);
POSE2=DATA(4:6);
POSE3=DATA(7:9);
POSE4=DATA(10:12);

POSES={POSE1,POSE2,POSE3,POSE4};
POSEi=POSES{i}; %determino el i robot (mismo algoritmo todos los robots)

POSEsorted=POSES;
for k=1:n
    POSEsorted{k}=POSES{I(k)};  
end 

%% Flocking
POSE_lead=POSEsorted{1};
x=zeros(1,n);
y=zeros(1,n);
theta=zeros(1,n);

x(1)=POSE_lead(1);
y(1)=POSE_lead(2);
theta(1)=POSE_lead(3);
xd=x(1);
yd=y(1);

for k=2:n
    POSE_current=POSEsorted{k};
    theta(k)=POSE_current(3);
    
    x(k)=x(k-1)+l*sin(theta(k-1)-theta_n);
    y(k)=y(k-1)+l*cos(theta(k-1)-theta_n);
end    
if i==I(1)
   way=WAY;
else
   for k=2:n
       if I(k)==i
          xd=x(k);
          yd=y(k);
          break;
       else
          xd=xd;
          yd=yd;
       end    
   end    
    %envio way para pure_pursuit
   way=WAY; 
   for k=1:kw
      if k<kw
        way(k,1)= POSEi(1);
        way(k,2)= POSEi(2);
      else
        way(k,1)= xd;
        way(k,2)= yd;   
      end
   end
end

== matlab function Four_Robots_Swarm/Swarm/TurtleBot3/selector ==
  data: sel input; way output; way_swap input; way_aggre input; way_flocking input
function way = fcn(sel,way_swap,way_aggre,way_flocking)
if sel==0
    way=way_swap;
elseif sel==1
    way=way_aggre;
elseif sel==2
    way=way_flocking;   
else
    way=way_swap;    
end

== matlab function Four_Robots_Swarm/Swarm/TurtleBot1/ Avoiding Obstacles/Path Following/Compute Angular Velocity ==
  data: steeringDir input; w output; wMax input
function w = exampleHelperComputeAngularVelocity(steeringDir, wMax)
%EXAMPLEHELPERCOMPUTEANGULARVELOCITY Compute angular velocity
%   W = exampleHelperComputeAngularVelocity(STEERINGDIR)
%   returns the angular velocity W for a differential drive robot in radians
%   per second for a given steering direction STEERINGDIR in the robot's
%   coordinate frame in radians.
%
%   W = exampleHelperComputeAngularVelocity(STEERINGDIR, WMAX)
%   returns the angular velocity W for a differential drive robot in radians
%   per second for a given steering direction STEERINGDIR in the robot's
%   coordinate frame in radians and maximum angular velocity WMAX in
%   radians per second. The output angular velocity is saturated based on
%   the WMAX.
%
%   Example:
%       
%       w = exampleHelperComputeAngularVelocity(0.2, 1);

% Copyright 2015 The MathWorks, Inc.

%#codegen
%#ok<*EMCA>

% Allow variable input arguments
if nargin == 1   
    wMax = inf;
end

validateattributes(steeringDir, {'double'},{'real'},...
    'exampleHelperComputeAngularVelocity', 'STEERINGDIR', 1);
validateattributes(wMax, {'double'},{'real', 'positive'},...
    'exampleHelperComputeAngularVelocity', 'WMAX', 2);

% Computing in robot's coordinate frame
curPose = [0 0 0];

% The following computation is similar to robotics.PurePursuit
lookaheadPoint = [cos(steeringDir), sin(steeringDir)];
slope = atan2((lookaheadPoint(2) - curPose(2)), ...
    (lookaheadPoint(1) - curPose(1)));
alpha = angdiff(curPose(3), slope);

% Angular velocity command for a differential drive robot is
% equal to the desired curvature to be followed by the robot.

w = (2*sin(alpha));

% Pick a constant rotation when robot is facing in the opposite
% direction of the path
if abs(abs(alpha) - pi) < 1e-12
    w = sign(w)*1;
end

if abs(w) > wMax
    w = sign(w)*wMax;
end

end

== matlab function Four_Robots_Swarm/Swarm/TurtleBot4/MATLAB Function2 ==
  data: p_i input; p_f input; way output
function way = fcn(p_i,p_f)
way=[p_i(1),p_i(2) ;p_f(1),p_f(2)];

== matlab function Four_Robots_Swarm/Swarm/TurtleBot4/Subsystem/Enabled Subsystem/MATLAB Function2 ==
  data: WAY input; DATA input; I output
function I  = fcn(WAY,DATA)
n=4;
POSE1=DATA(1:3);
POSE2=DATA(4:6);
POSE3=DATA(7:9);
POSE4=DATA(10:12);

POSES={POSE1,POSE2,POSE3,POSE4};

%% Cálculo distancias robots- origen trayectoria
xway=WAY(1,1);
yway=WAY(1,2);
d=zeros(1,n);
for j=1:n
  POSEj=POSES{j};  
  d(j)=sqrt((xway-POSEj(1))^2+(yway-POSEj(2))^2);  
end
%% Determino orden robots
[~,I]=sort(d);

== matlab function Four_Robots_Swarm/Swarm/TurtleBot4/Subsystem/MATLAB Function1 ==
  data: WAY input; DATA input; way output double; i input; I input; l input; theta_n input
function way = fcn(WAY,DATA,i,I,l,theta_n)
n=4;
kw=size(WAY,1);
POSE1=DATA(1:3);
POSE2=DATA(4:6);
POSE3=DATA(7:9);
POSE4=DATA(10:12);

POSES={POSE1,POSE2,POSE3,POSE4};
POSEi=POSES{i}; %determino el i robot (mismo algoritmo todos los robots)

POSEsorted=POSES;
for k=1:n
    POSEsorted{k}=POSES{I(k)};  
end 

%% Flocking
POSE_lead=POSEsorted{1};
x=zeros(1,n);
y=zeros(1,n);
theta=zeros(1,n);

x(1)=POSE_lead(1);
y(1)=POSE_lead(2);
theta(1)=POSE_lead(3);
xd=x(1);
yd=y(1);

for k=2:n
    POSE_current=POSEsorted{k};
    theta(k)=POSE_current(3);
    
    x(k)=x(k-1)+l*sin(theta(k-1)-theta_n);
    y(k)=y(k-1)+l*cos(theta(k-1)-theta_n);
end    
if i==I(1)
   way=WAY;
else
   for k=2:n
       if I(k)==i
          xd=x(k);
          yd=y(k);
          break;
       else
          xd=xd;
          yd=yd;
       end    
   end    
    %envio way para pure_pursuit
   way=WAY; 
   for k=1:kw
      if k<kw
        way(k,1)= POSEi(1);
        way(k,2)= POSEi(2);
      else
        way(k,1)= xd;
        way(k,2)= yd;   
      end
   end
end

== matlab function Four_Robots_Swarm/Swarm/TurtleBot4/selector ==
  data: sel input; way output; way_swap input; way_aggre input; way_flocking input
function way = fcn(sel,way_swap,way_aggre,way_flocking)
if sel==0
    way=way_swap;
elseif sel==1
    way=way_aggre;
elseif sel==2
    way=way_flocking;   
else
    way=way_swap;    
end

== matlab function Four_Robots_Swarm/Joystick/Triggered Subsystem/MATLAB Function2 ==
  data: A input; modo output; B input; X input; Y input; mode input
function modo = fcn(A, B, X, Y, mode)
if A==1
modo=0;
elseif B==1
modo=1;
elseif Y==1
modo=2;
else
modo=mode;    
end

== matlab function Four_Robots_Swarm/Swarm/TurtleBot1/ Path following/ Extract Goal ==
  data: Waypoints input; Goal output
function Goal = extractGoal(Waypoints)
%#codegen
b = isnan(Waypoints);
[rows,~] = find(b);
ridx = setdiff(1:size(Waypoints,1), sort(rows));
Goal = [Waypoints(ridx(end), 1) Waypoints(ridx(end), 2)];

== matlab function Four_Robots_Swarm/Swarm/TurtleBot3/Inputs/MATLAB Function ==
  data: LaserScanMsg input; Ranges output; Angles output
function [Ranges, Angles] = ExtractRangeData(LaserScanMsg)
%#codegen

% Extract Range information
Ranges = double(LaserScanMsg.Ranges);

% Construct Angles vector using AngleMin and AngleIncrement from sensor
% reading.
angMin = double(LaserScanMsg.AngleMin);
angIncrement = double(LaserScanMsg.AngleIncrement);

numReadings = numel(Ranges);
rawAngles = angMin + (0:numReadings-1)' * angIncrement;

% Wrap the angles to the (-pi,pi] interval.
Angles = robotics.internal.wrapToPi(double(rawAngles));

== matlab function Four_Robots_Swarm/Swarm/TurtleBot1/Inputs/MATLAB Function ==
  data: LaserScanMsg input; Ranges output; Angles output
function [Ranges, Angles] = ExtractRangeData(LaserScanMsg)
%#codegen

% Extract Range information
Ranges = double(LaserScanMsg.Ranges);

% Construct Angles vector using AngleMin and AngleIncrement from sensor
% reading.
angMin = double(LaserScanMsg.AngleMin);
angIncrement = double(LaserScanMsg.AngleIncrement);

numReadings = numel(Ranges);
rawAngles = angMin + (0:numReadings-1)' * angIncrement;

% Wrap the angles to the (-pi,pi] interval.
Angles = robotics.internal.wrapToPi(double(rawAngles));

== matlab function Four_Robots_Swarm/Swarm/TurtleBot3/ Path following/ Extract Goal ==
  data: Waypoints input; Goal output
function Goal = extractGoal(Waypoints)
%#codegen
b = isnan(Waypoints);
[rows,~] = find(b);
ridx = setdiff(1:size(Waypoints,1), sort(rows));
Goal = [Waypoints(ridx(end), 1) Waypoints(ridx(end), 2)];

== matlab function Four_Robots_Swarm/Swarm/TurtleBot1/Inputs/quad2eul ==
  data: X input; Yaw output; Y input; Z input; W input
function Yaw = quat2eulBlk(X, Y, Z, W)
%#codegen

eularAngles = quat2eul([W, X, Y, Z]);
Yaw = eularAngles(1);

== matlab function Four_Robots_Swarm/Swarm/TurtleBot2/ Avoiding Obstacles/Path Following/Compute Angular Velocity ==
  data: steeringDir input; w output; wMax input
function w = exampleHelperComputeAngularVelocity(steeringDir, wMax)
%EXAMPLEHELPERCOMPUTEANGULARVELOCITY Compute angular velocity
%   W = exampleHelperComputeAngularVelocity(STEERINGDIR)
%   returns the angular velocity W for a differential drive robot in radians
%   per second for a given steering direction STEERINGDIR in the robot's
%   coordinate frame in radians.
%
%   W = exampleHelperComputeAngularVelocity(STEERINGDIR, WMAX)
%   returns the angular velocity W for a differential drive robot in radians
%   per second for a given steering direction STEERINGDIR in the robot's
%   coordinate frame in radians and maximum angular velocity WMAX in
%   radians per second. The output angular velocity is saturated based on
%   the WMAX.
%
%   Example:
%       
%       w = exampleHelperComputeAngularVelocity(0.2, 1);

% Copyright 2015 The MathWorks, Inc.

%#codegen
%#ok<*EMCA>

% Allow variable input arguments
if nargin == 1   
    wMax = inf;
end

validateattributes(steeringDir, {'double'},{'real'},...
    'exampleHelperComputeAngularVelocity', 'STEERINGDIR', 1);
validateattributes(wMax, {'double'},{'real', 'positive'},...
    'exampleHelperComputeAngularVelocity', 'WMAX', 2);

% Computing in robot's coordinate frame
curPose = [0 0 0];

% The following computation is similar to robotics.PurePursuit
lookaheadPoint = [cos(steeringDir), sin(steeringDir)];
slope = atan2((lookaheadPoint(2) - curPose(2)), ...
    (lookaheadPoint(1) - curPose(1)));
alpha = angdiff(curPose(3), slope);

% Angular velocity command for a differential drive robot is
% equal to the desired curvature to be followed by the robot.

w = (2*sin(alpha));

% Pick a constant rotation when robot is facing in the opposite
% direction of the path
if abs(abs(alpha) - pi) < 1e-12
    w = sign(w)*1;
end

if abs(w) > wMax
    w = sign(w)*wMax;
end

end

== matlab function Four_Robots_Swarm/Swarm/TurtleBot2/ Path following/ Extract Goal ==
  data: Waypoints input; Goal output
function Goal = extractGoal(Waypoints)
%#codegen
b = isnan(Waypoints);
[rows,~] = find(b);
ridx = setdiff(1:size(Waypoints,1), sort(rows));
Goal = [Waypoints(ridx(end), 1) Waypoints(ridx(end), 2)];

== matlab function Four_Robots_Swarm/Swarm/TurtleBot2/Inputs/MATLAB Function ==
  data: LaserScanMsg input; Ranges output; Angles output
function [Ranges, Angles] = ExtractRangeData(LaserScanMsg)
%#codegen

% Extract Range information
Ranges = double(LaserScanMsg.Ranges);

% Construct Angles vector using AngleMin and AngleIncrement from sensor
% reading.
angMin = double(LaserScanMsg.AngleMin);
angIncrement = double(LaserScanMsg.AngleIncrement);

numReadings = numel(Ranges);
rawAngles = angMin + (0:numReadings-1)' * angIncrement;

% Wrap the angles to the (-pi,pi] interval.
Angles = robotics.internal.wrapToPi(double(rawAngles));
